simulink model "SS_Part6"  (R2024b)
settings: Solver=ode45  StartTime=0.0  StopTime=tstop  FixedStep=10  RelTol=1e-6  AbsTol=1e-8
values from neighbouring files (symbols this model uses):
  C_b_wi = cat(3, C_b_w1, C_b_w2, C_b_w3)    [SS_Part6Script.m]
  I_tot = I_sc + I_RWsum    [SS_Part6Script.m]
  I_wi = cat(3, I_w1, I_w2, I_w3)    [SS_Part6Script.m]
  Kd = J/ts    [Part5_TorqueFreeMotion_SS.m]    (also in Part_5_ORR.m = J*eye(3)*2*zeta*wn; SS_Part6Script.m = 2*zeta*wn*I_tot)
  Kp = zeros(3)    [Part5_TorqueFreeMotion_SS.m]    (also in Part_5_ORR.m = 2*J*eye(3)*wn^2; SS_Part6Script.m = 2*wn^2*I_tot)
  orbParams = getMoreOrbitalParams(hmag, ecc, TA, raan, inc, argp, muE)    [Part2_TorqueFreeMotion.m]    (also in Part2_TorqueFreeMotion_SS.m; Part5_TorqueFreeMotion_SS.m; SS_Part6Script.m)
  q0_b_ECI = DCM_to_quat(C_b_ECI_0)    [SS_Part6Script.m]
  q_C = [0; 0; 0; 1]    [Part5_TorqueFreeMotion_SS.m]    (also in SS_Part6Script.m = [0;0;0;1])
  w0_b_ECI = [0.001; -0.001; 0.002]    [SS_Part6Script.m]
  w0_wi_ECI = zeros(num_wheels,1)    [SS_Part6Script.m]
settings Model: Creator=emehiel  LastModifiedBy=dstan
settings SolverCC: AlgebraicLoopSolver=TrustRegion
settings DebuggingCC: UnconnectedInputMsg=warning  UnconnectedOutputMsg=warning  UnconnectedLineMsg=warning
settings ModelReferenceCC: EnableRefExpFcnMdlSchedulingChecks=on
settings RTWCC: GPUComputeCapability=3.5

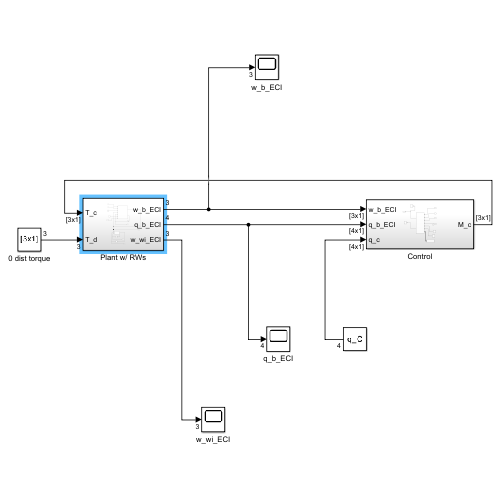
[thumbnail: Simulink's stored preview of the top-level diagram]
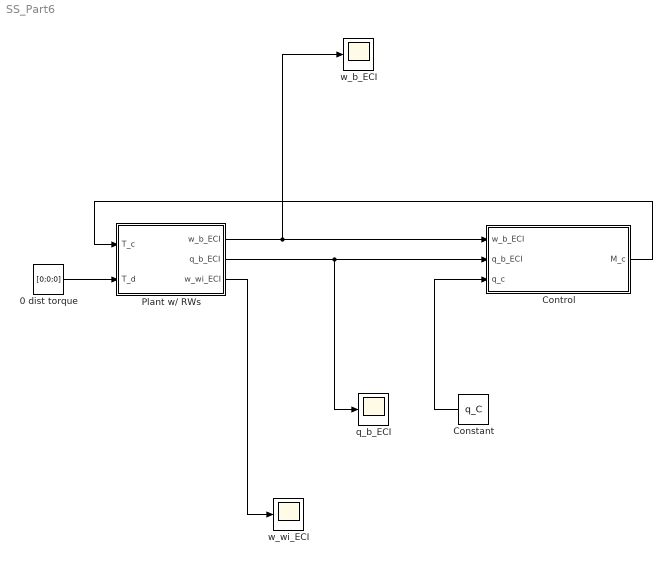
== system SS_Part6 ==
  0 dist torque : Constant  Value=[0;0;0]
  Constant : Constant  Value=q_C
  Control : Subsystem
  Plant w/ RWs : Subsystem
  q_b_ECI : Scope
  w_b_ECI : Scope
  w_wi_ECI : Scope
  wires:
  Plant w/ RWs/2(q_b_ECI) -> Control/2(q_b_ECI), q_b_ECI/1
  Constant/1 -> Control/3(q_c)
  Control/1(M_c) -> Plant w/ RWs/1(T_c)
  Plant w/ RWs/3(w_wi_ECI) -> w_wi_ECI/1
  Plant w/ RWs/1(w_b_ECI) -> Control/1(w_b_ECI), w_b_ECI/1
  0 dist torque/1 -> Plant w/ RWs/2(T_d)

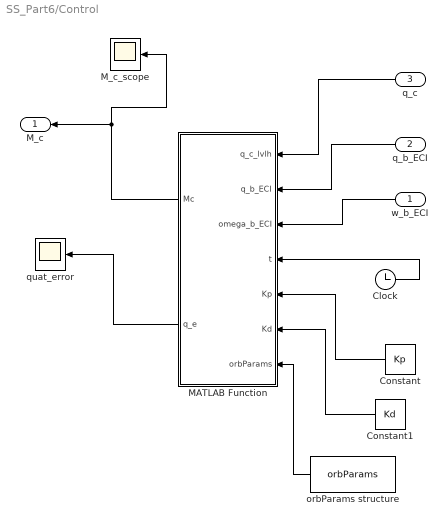
== system SS_Part6/Control ==
  w_b_ECI : Inport  PortDimensions=[3 1]
  q_b_ECI : Inport  Port=2  PortDimensions=[4 1]
  q_c : Inport  Port=3  PortDimensions=[4 1]
  Clock : Clock
  Constant : Constant  Value=Kp
  Constant1 : Constant  Value=Kd
  MATLAB Function : MATLAB Function  TreatAsAtomicUnit=on
  M_c_scope : Scope
  orbParams structure : Constant  Value=orbParams  OutDataTypeStr=Bus: slBus1
  quat_error : Scope
  M_c : Outport  PortDimensions=[3 1]  VectorParamsAs1DForOutWhenUnconnected=off
  wires:
  MATLAB Function/1(Mc) -> M_c_scope/1, M_c/1
  q_c/1 -> MATLAB Function/1(q_c_lvlh)
  w_b_ECI/1 -> MATLAB Function/3(omega_b_ECI)
  q_b_ECI/1 -> MATLAB Function/2(q_b_ECI)
  Constant/1 -> MATLAB Function/5(Kp)
  MATLAB Function/2(q_e) -> quat_error/1
  Constant1/1 -> MATLAB Function/6(Kd)
  Clock/1 -> MATLAB Function/4(t)
  orbParams structure/1 -> MATLAB Function/7(orbParams)

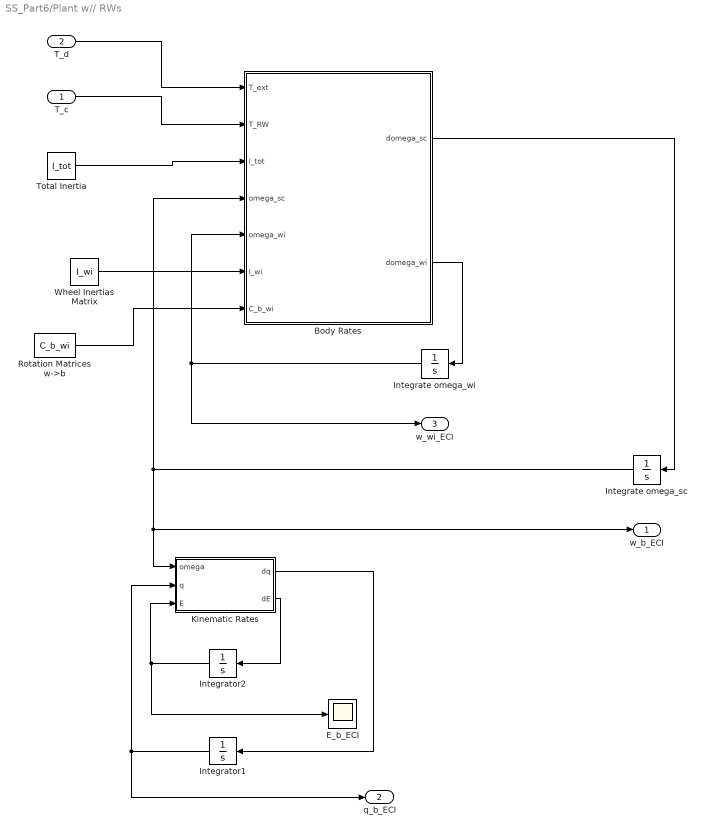
== system SS_Part6/Plant w// RWs ==
  T_c : Inport
  T_d : Inport  Port=2
  Body Rates : MATLAB Function  TreatAsAtomicUnit=on
  E_b_ECI : Scope
  Integrate omega_sc : Integrator  InitialCondition=w0_b_ECI
  Integrate omega_wi : Integrator  InitialCondition=w0_wi_ECI
  Integrator1 : Integrator  InitialCondition=q0_b_ECI
  Integrator2 : Integrator  InitialCondition=[0;0;0]
  Kinematic Rates : MATLAB Function  TreatAsAtomicUnit=on
  Rotation Matrices w->b : Constant  Value=C_b_wi
  Total Inertia : Constant  Value=I_tot
  Wheel Inertias Matrix : Constant  Value=I_wi
  w_b_ECI : Outport
  q_b_ECI : Outport  Port=2
  w_wi_ECI : Outport  Port=3
  wires:
  Integrate omega_sc/1 -> Body Rates/4(omega_sc), Kinematic Rates/1(omega), w_b_ECI/1
  Integrator2/1 -> E_b_ECI/1, Kinematic Rates/3(E)
  Kinematic Rates/1(dq) -> Integrator1/1
  Integrator1/1 -> q_b_ECI/1, Kinematic Rates/2(q)
  Body Rates/1(domega_sc) -> Integrate omega_sc/1
  Total Inertia/1 -> Body Rates/3(I_tot)
  Kinematic Rates/2(dE) -> Integrator2/1
  Wheel Inertias Matrix/1 -> Body Rates/6(I_wi)
  Rotation Matrices w->b/1 -> Body Rates/7(C_b_wi)
  Body Rates/2(domega_wi) -> Integrate omega_wi/1
  Integrate omega_wi/1 -> w_wi_ECI/1, Body Rates/5(omega_wi)
  T_c/1 -> Body Rates/2(T_RW)
  T_d/1 -> Body Rates/1(T_ext)

== matlab function SS_Part6/Plant w// RWs/Kinematic Rates ==
  data: omega input; q input; dq output; E input; dE output
function [dq, dE] = kinematics(omega, q, E)
% column vecs
omega = omega(:);
q = q(:);
E = E(:);

% unpack euler angles
phi = E(1);
theta = E(2);
psi = E(3);

% unpack quat
eps = q(1:3);
eta = q(4);

% euler derivative
B = [1, sin(phi)*tan(theta),  cos(phi)*tan(theta);
     0, cos(phi),            -sin(phi);
     0, sin(phi)/cos(theta),  cos(phi)/cos(theta)];

dE = B * omega;

% quat derivative
dq = zeros(4,1);
dq(1:3) = 0.5 * ((eta*eye(3) + skew(eps)) * omega);
dq(4)   = -0.5 * (eps.' * omega);

end

== matlab function SS_Part6/Plant w// RWs/Body Rates ==
  data: T_ext input; T_RW input; I_tot input; domega_sc output; omega_sc input; omega_wi input; I_wi input; C_b_wi input; domega_wi output
function [domega_sc, domega_wi]= dynamics(T_ext, T_RW, I_tot, omega_sc, omega_wi, I_wi, C_b_wi)

% Convert to matlab column vectors simulink is being weird with shape reqs?
T_ext = reshape(T_ext, 3, 1);
T_RW = reshape(T_RW, 3, 1);
omega_sc = reshape(omega_sc, 3, 1);

num_wheels = size(I_wi, 3);
omega_wi = reshape(omega_wi, num_wheels, 1);

% get angular momentums
h_sc = I_tot*omega_sc;

h_RW_sum = zeros(3,1);
for i = 1:num_wheels
    I_si = I_wi(1,1,i);
    % wheel angular momentum is only along wheel-frame x-axis
    h_wheel_i = [I_si*omega_wi(i); 0; 0];

    % rotate wheel angular momentum into body frame
    h_RW_sum = h_RW_sum + C_b_wi(:,:,i)*h_wheel_i;
end
h_RW = h_RW_sum;

% total torque on sc
T_tot = T_ext + T_RW;

% time derivative of sc ang velo
domega_sc = I_tot \ (T_tot - skew(omega_sc)*h_sc - skew(omega_sc)*h_RW);

% time derivative of wheel speeds
% one scalar angular acceleration per wheel
domega_wi = zeros(num_wheels,1);

for i = 1:num_wheels
    I_si = I_wi(1,1,i);

    % wheel spin axis expressed in body frame
    spin_axis_body = C_b_wi(:,:,i)*[1;0;0];

    % project commanded spacecraft torque onto that wheel axis
    T_sc_i = dot(T_RW, spin_axis_body);

    % wheel torque is equal and opposite
    domega_wi(i) = -T_sc_i/I_si;
end
end

== matlab function SS_Part6/Control/MATLAB Function ==
  data: q_c_lvlh input; Mc output; q_b_ECI input; omega_b_ECI input; t input; Kp input; Kd input; q_e output; orbParams input
function [Mc,q_e] = control_law_lvlh(q_c_lvlh, q_b_ECI, omega_b_ECI, t, Kp, Kd, orbParams)

% column vecs
q_c_lvlh   = q_c_lvlh(:);
q_b_ECI    = q_b_ECI(:);
omega_b_ECI = omega_b_ECI(:);

% get current orbit true anomaly
TA_k = orbParams.TA + orbParams.n*t;

muE = orbParams.mu;

% current orbit state
[r_ECI, v_ECI] = coesToState(orbParams.hmag, ...
                             orbParams.ecc, ...
                             TA_k, ...
                             orbParams.raan, ...
                             orbParams.inc, ...
                             orbParams.argp, ...
                             muE);

% LVLH to ECI DCM
C_LVLH_ECI = LVLH_from_ECI(r_ECI, v_ECI);

% body to ECI DCM from current quaternion
C_b_ECI = quat_to_DCM(q_b_ECI);

% body to LVLH DCM
C_b_LVLH = C_b_ECI * C_LVLH_ECI';

% current body-to-LVLH quaternion
q_b_LVLH = DCM_to_quat(C_b_LVLH);

% shortest quaternion direction
if q_b_LVLH(4) < 0
    q_b_LVLH = -q_b_LVLH;
end

% LVLH angular velocity wrt ECI, expressed in ECI
h_ECI = cross(r_ECI, v_ECI);
omega_LVLH_ECI_ECI = h_ECI / norm(r_ECI)^2;

% LVLH angular velocity wrt ECI, expressed in body
omega_LVLH_ECI_b = C_b_ECI * omega_LVLH_ECI_ECI;

% spacecraft angular velocity wrt LVLH, expressed in body
omega_b_LVLH = omega_b_ECI - omega_LVLH_ECI_b;

% quaternion error relative to LVLH command
q_e = quatMult(quatConjugate(q_c_lvlh), q_b_LVLH);

% use short way around
if q_e(4) < 0
    q_e = -q_e;
end

% full state feedback in body frame
Mc = -Kp*q_e(1:3) - Kd*omega_b_LVLH;

end
